simulink model "magball"  (R2023b)
settings: Solver=VariableStepAuto  StartTime=0.0  StopTime=1  RelTol=1e-3
undefined symbols (not defined in the file): g, L, M, R, y0
settings Model: Creator=cr  LastModifiedBy=cr

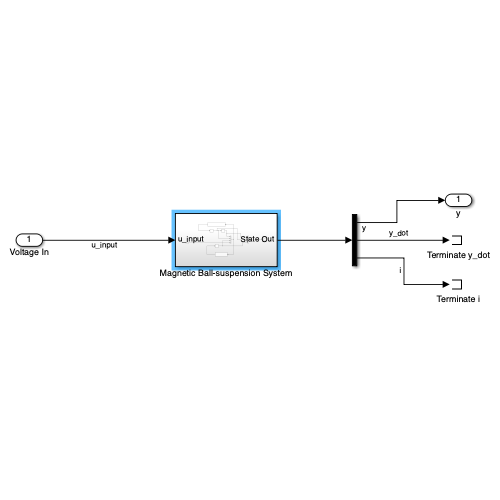
[thumbnail: Simulink's stored preview of the top-level diagram]
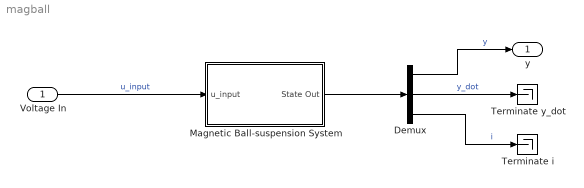
== system magball ==
  Voltage In : Inport
  Demux : Demux  Outputs=3
  Magnetic Ball-suspension System : Subsystem
  Terminate i : Terminator
  Terminate y_dot : Terminator
  y : Outport
  wires:
  Voltage In/1 -> Magnetic Ball-suspension System/1(u_input)  "u_input"
  Magnetic Ball-suspension System/1(State Out) -> Demux/1
  Demux/2 -> Terminate y_dot/1  "y_dot"
  Demux/1 -> y/1  "y"
  Demux/3 -> Terminate i/1  "i"

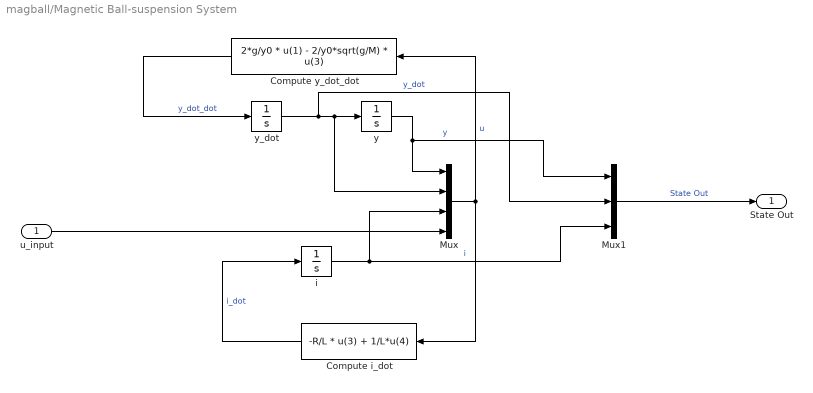
== system magball/Magnetic Ball-suspension System ==
  u_input : Inport
  Compute i_dot : Fcn  Expr=-R/L * u(3) + 1/L*u(4)
  Compute y_dot_dot : Fcn  Expr=2*g/y0 * u(1) - 2/y0*sqrt(g/M) * u(3)
  Mux : Mux
  Mux1 : Mux  Inputs=3
  i : Integrator
  y : Integrator
  y_dot : Integrator
  State Out : Outport
  wires:
  Mux1/1 -> State Out/1  "State Out"
  Compute i_dot/1 -> i/1  "i_dot"
  y_dot/1 -> Mux1/2, Mux/2, y/1  "y_dot"
  Mux/1 -> Compute i_dot/1, Compute y_dot_dot/1  "u"
  i/1 -> Mux1/3, Mux/3  "i"
  u_input/1 -> Mux/4
  Compute y_dot_dot/1 -> y_dot/1  "y_dot_dot"
  y/1 -> Mux1/1, Mux/1  "y"
